simulink subsystem "GenericScanner"  (R2025b)
settings: Solver=VariableStepAuto  StartTime=0.0  StopTime=10.0  RelTol=1e-3
values from neighbouring files (symbols this model uses):
  m = min(v)    [run_loader_scanner_model_multi_stress_v1_2_final_verified.m]    (also in run_slide_model_daily_scenarios_v2.m; run_slide_model_daily_scenarios_v2_scannerbank_v2.m)
  n = round(v(end))    [run_loader_scanner_model_multi_stress_v1_2_final_verified.m]    (also in run_slide_model_daily_scenarios_v2.m = numel(logs); run_slide_model_daily_scenarios_v2_scannerbank_v2.m)
undefined symbols (not defined in the file or in its folder): RackLoaded
libraries: simulink x5
settings Model: Creator=bayes  LastModifiedBy=bayes

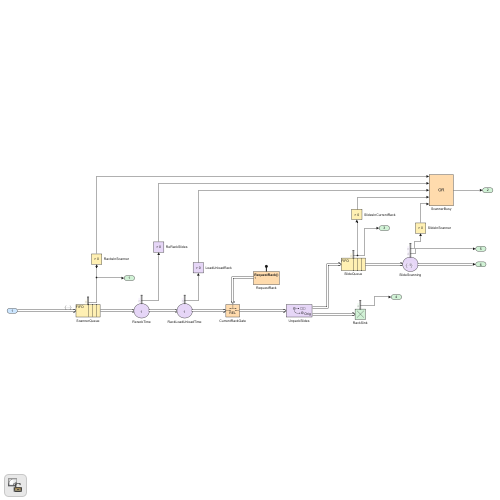
[thumbnail: Simulink's stored preview of the top-level diagram]
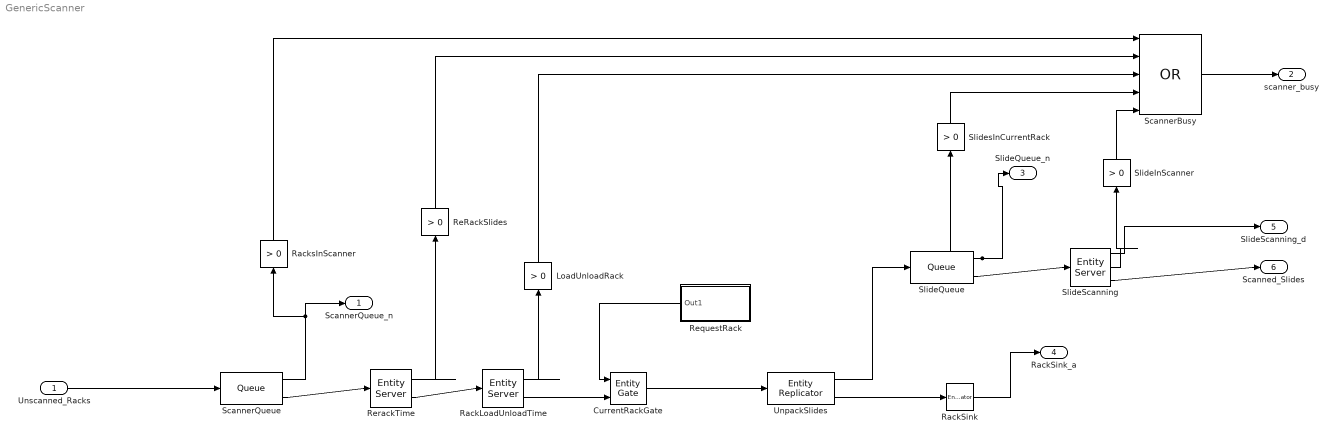
== system GenericScanner ==
  Unscanned_Racks : Inport
  CurrentRackGate : EntityGate  InputPortMessageModes=m,m  OutputPortMessageModes=m  OperatingMode=Release gate  OpenGateAtSimulationStart=on
  LoadUnloadRack : simulink/Logic and Bit Operations/Compare To Zero  relop=>  OutDataTypeStr=boolean
  RackLoadUnloadTime : EntityServer  InputPortMessageModes=m  OutputPortMessageModes=n,m  Capacity=1  ServiceTimeValue=Scanner_RackLoadTime  NumberEntitiesInBlock=on
      settings: OutputPortMap=o1,o9
  RackSink : EntityTerminator  InputPortMessageModes=m  NumberEntitiesArrived=on
      settings: OutputPortMap=o0
  RacksInScanner : simulink/Logic and Bit Operations/Compare To Zero  relop=>  OutDataTypeStr=boolean
  ReRackSlides : simulink/Logic and Bit Operations/Compare To Zero  relop=>  OutDataTypeStr=boolean
  RequestRack : Subsystem  TreatAsAtomicUnit=on
  RerackTime : EntityServer  InputPortMessageModes=m  OutputPortMessageModes=n,m  Capacity=1  ServiceTimeValue=Scanner_RerackTime  NumberEntitiesInBlock=on
      settings: OutputPortMap=o1,o9
  ScannerBusy : Logic  Operator=OR  Inputs=5  AllPortsSameDT=off  OutDataTypeStr=boolean
  ScannerQueue : Queue  InputPortMessageModes=m  OutputPortMessageModes=n,m  Capacity=Scanner_RackQueueSize  EntryAction=RackLoaded();  NumberEntitiesInBlock=on
      settings: OutputPortMap=o1,o5
  SlideInScanner : simulink/Logic and Bit Operations/Compare To Zero  relop=>  OutDataTypeStr=boolean
  SlideQueue : Queue  InputPortMessageModes=m  OutputPortMessageModes=n,m  Capacity=Scanner_SlideQueueSize  NumberEntitiesInBlock=on
      settings: OutputPortMap=o1,o5
  SlideScanning : EntityServer  InputPortMessageModes=m  OutputPortMessageModes=n,n,m  Capacity=1  ServiceTimeSource=MATLAB action  ServiceTimeValue=Scanner_SlideScanTime  ServiceTimeAction=dt = exp(ScanTime_Mu + ScanTime_Sigma * randn(1));  ServiceCompleteAction=|  NumberEntitiesDeparted=on  NumberEntitiesInBlock=on
      | persistent scannedCount;
      | 
      | if isempty(scannedCount)
      |     scannedCount = 0;
      | end
      | 
      | scannedCount = scannedCount + 1;
      | 
      | if scannedCount >= entity.SlideCount
      |     scannedCount = 0;
      |     RequestRack();
      | end
      settings: OutputPortMap=o0,o1,o9
  SlidesInCurrentRack : simulink/Logic and Bit Operations/Compare To Zero  relop=>  OutDataTypeStr=boolean
  UnpackSlides : EntityReplicator  InputPortMessageModes=m  OutputPortMessageModes=m,m  ReplicasDepartFrom=Single output port  ReplicationAmountSource=Attribute  ReplicateAttributeName=SlideCount  HoldOriginalEntityUntilAllReplicasDepart=on
  ScannerQueue_n : Outport
  scanner_busy : Outport  Port=2
  SlideQueue_n : Outport  Port=3
  RackSink_a : Outport  Port=4
  SlideScanning_d : Outport  Port=5
  Scanned_Slides : Outport  Port=6
  wires:
  ScannerQueue/1 -> RacksInScanner/1, ScannerQueue_n/1
  UnpackSlides/1 -> SlideQueue/1
  UnpackSlides/2 -> RackSink/1
  RequestRack/1(Out1) -> CurrentRackGate/1
  SlideQueue/2 -> SlideScanning/1
  RackLoadUnloadTime/2 -> CurrentRackGate/2
  ScannerQueue/2 -> RerackTime/1
  SlideScanning/1 -> SlideScanning_d/1
  RerackTime/2 -> RackLoadUnloadTime/1
  CurrentRackGate/1 -> UnpackSlides/1
  RackSink/1 -> RackSink_a/1
  SlideScanning/3 -> Scanned_Slides/1
  SlideQueue/1 -> SlideQueue_n/1, SlidesInCurrentRack/1
  Unscanned_Racks/1 -> ScannerQueue/1
  RackLoadUnloadTime/1 -> LoadUnloadRack/1
  RerackTime/1 -> ReRackSlides/1
  SlidesInCurrentRack/1 -> ScannerBusy/4
  LoadUnloadRack/1 -> ScannerBusy/3
  ReRackSlides/1 -> ScannerBusy/2
  RacksInScanner/1 -> ScannerBusy/1
  ScannerBusy/1 -> scanner_busy/1
  SlideInScanner/1 -> ScannerBusy/5
  SlideScanning/2 -> SlideInScanner/1

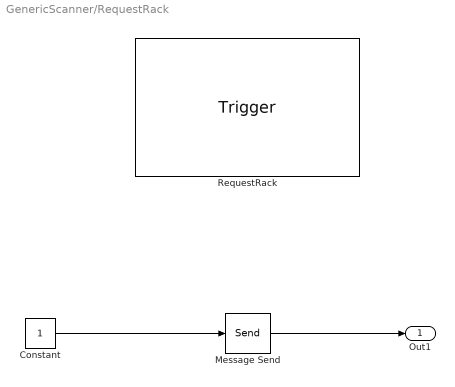
== system GenericScanner/RequestRack ==
  RequestRack : TriggerPort  TriggerType=function-call  IsSimulinkFunction=on  FunctionName=RequestRack  FunctionVisibility=scoped  VariantControl=(inherit)
  Constant : Constant
  Message Send : Send  OutputPortMessageModes=m
  Out1 : Outport
  wires:
  Message Send/1 -> Out1/1
  Constant/1 -> Message Send/1
